simulink model "YawModel_R3 (1)"  (R2013a)
settings: Solver=ode45  StartTime=0.0  StopTime=30  RelTol=1e-3
values from neighbouring files (symbols this model uses):
  D = 4.45306861536e-07    [Parameters.mat]
  I_Psi = 0.236966962973    [Parameters.mat]
  J = 8e-08    [Parameters.mat]
  Kd_Yaw = K*T_d    [Yaw_PID.m]
  Ki_Yaw = K/T_I    [Yaw_PID.m]
  Kp_Yaw = K    [Yaw_PID.m]
  Kw = 501.513336009    [Parameters.mat]
  Motor_TimeConstant = 0.07    [Parameters.mat]
  omega_0 = 520    [Yaw_PID.m]
  Speed_yIntercept = -347.939581678    [Parameters.mat]
libraries: simulink x2
settings Model: Creator=Ross  LastModifiedBy=Ross

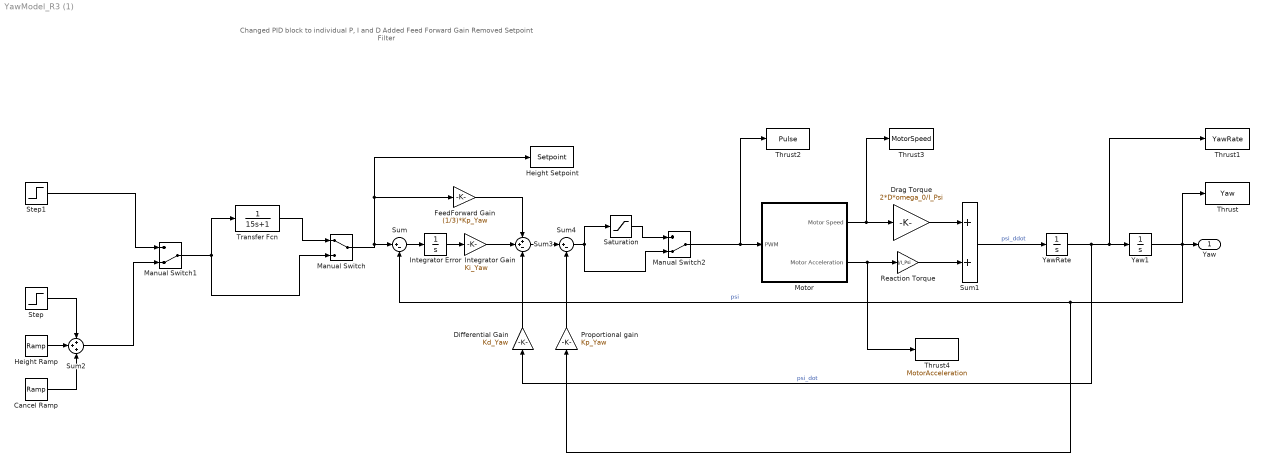
== system YawModel_R3 (1) ==
  note: Changed PID block to individual P, I and D
      | Added Feed Forward Gain
      | Removed Setpoint Filter
  Cancel Ramp : simulink/Sources/Ramp  slope=-0.5  start=5  X0=0
  Differential Gain : Gain  Gain=Kd_Yaw
  Drag Torque : Gain  Gain=2*D*omega_0/I_Psi
  FeedForward Gain : Gain  Gain=(1/3)*Kp_Yaw
  Height Ramp : simulink/Sources/Ramp  slope=0.5  start=1  X0=0
  Height Setpoint : ToWorkspace  VariableName=Setpoint  SampleTime=-1  SaveFormat=Timeseries
  Integrator Error : Integrator
  Integrator Gain : Gain  Gain=Ki_Yaw
  Manual Switch : ManualSwitch
  Manual Switch1 : ManualSwitch  CurrentSetting=0
  Manual Switch2 : ManualSwitch  CurrentSetting=0
  Motor : Subsystem
  Proportional gain : Gain  Gain=Kp_Yaw
  Reaction Torque : Gain  Gain=J/I_Psi
  Saturation : Saturate  UpperLimit=2  LowerLimit=-2
  Step : Step  Time=10  SampleTime=0
  Step1 : Step  SampleTime=0
  Sum : Sum  Inputs=|+-
  Sum1 : Sum
  Sum2 : Sum  Inputs=+++
  Sum3 : Sum  Inputs=++-
  Sum4 : Sum  Inputs=|+-
  Thrust : ToWorkspace  VariableName=Yaw  SampleTime=-1  SaveFormat=Timeseries
  Thrust1 : ToWorkspace  VariableName=YawRate  SampleTime=-1  SaveFormat=Timeseries
  Thrust2 : ToWorkspace  VariableName=Pulse  SampleTime=-1  SaveFormat=Timeseries
  Thrust3 : ToWorkspace  VariableName=MotorSpeed  SampleTime=-1  SaveFormat=Timeseries
  Thrust4 : ToWorkspace  VariableName=MotorAcceleration  SampleTime=-1  SaveFormat=Timeseries
  Transfer Fcn : TransferFcn  Denominator=[15 1]
  Yaw1 : Integrator  LowerSaturationLimit=0
  YawRate : Integrator
  Yaw : Outport
  wires:
  Yaw1/1 -> Proportional gain/1, Sum/2, Thrust/1, Yaw/1  "psi"
  YawRate/1 -> Differential Gain/1, Thrust1/1, Yaw1/1  "psi_dot"
  Sum1/1 -> YawRate/1  "psi_ddot"
  Motor/2(Motor Acceleration) -> Thrust4/1, Reaction Torque/1
  Drag Torque/1 -> Sum1/1
  Reaction Torque/1 -> Sum1/2
  Step/1 -> Sum2/1
  Height Ramp/1 -> Sum2/2
  Cancel Ramp/1 -> Sum2/3
  Sum/1 -> Integrator Error/1
  Motor/1(Motor Speed) -> Drag Torque/1, Thrust3/1
  Integrator Error/1 -> Integrator Gain/1
  Sum3/1 -> Sum4/1
  Proportional gain/1 -> Sum4/2
  Differential Gain/1 -> Sum3/3
  Integrator Gain/1 -> Sum3/2
  FeedForward Gain/1 -> Sum3/1
  Manual Switch/1 -> FeedForward Gain/1, Height Setpoint/1, Sum/1
  Transfer Fcn/1 -> Manual Switch/1
  Manual Switch1/1 -> Transfer Fcn/1, Manual Switch/2
  Sum2/1 -> Manual Switch1/2
  Step1/1 -> Manual Switch1/1
  Sum4/1 -> Saturation/1, Manual Switch2/2
  Manual Switch2/1 -> Thrust2/1, Motor/1(PWM)
  Saturation/1 -> Manual Switch2/1

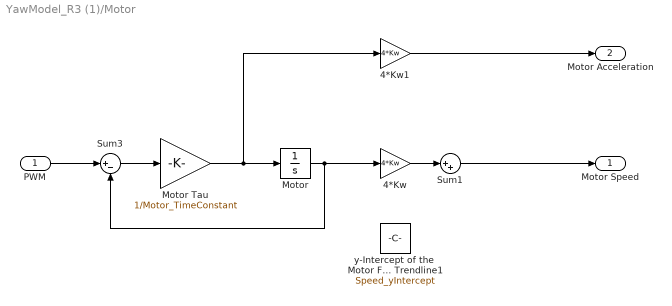
== system YawModel_R3 (1)/Motor ==
  PWM : Inport
  4*Kw : Gain  Gain=4*Kw
  4*Kw1 : Gain  Gain=4*Kw
  Motor : Integrator
  Motor Tau : Gain  Gain=1/Motor_TimeConstant
  Sum1 : Sum  Inputs=|++
  Sum3 : Sum  Inputs=|+-
  y-Intercept of the  Motor Forc Trendline1 : Constant  Value=Speed_yIntercept
  Motor Speed : Outport
  Motor Acceleration : Outport  Port=2
  wires:
  Motor Tau/1 -> 4*Kw1/1, Motor/1
  Motor/1 -> 4*Kw/1, Sum3/2
  PWM/1 -> Sum3/1
  Sum3/1 -> Motor Tau/1
  4*Kw/1 -> Sum1/1
  Sum1/1 -> Motor Speed/1
  4*Kw1/1 -> Motor Acceleration/1
